simulink model "motor_kit_sim_20MHz"  (R2024a)
settings: Solver=VariableStepAuto  StartTime=0.0  StopTime=10*62.5E-6  RelTol=1e-3  EnableMultiTasking=on
PreLoadFcn:
  | setup_motor_kit_sim_20MHz;
InitFcn:
  | setup_motor_kit_sim_20MHz;
values from neighbouring files (symbols this model uses):
  DSPBASampleTime = 0.05e-6    (= 5e-08)    [setup_motor_kit_sim_20MHz.m]
  wordLength = 16    [setup_motor_kit_sim_20MHz.m]
undefined symbols (not defined in the file or in its folder): AdvDSPBChannelOutDisplay, dpoly, dspba_internal_get_channel_ports, evalAionMaskParam, latency, primtype, value, x
libraries: DSPBAPrim x317, DSPBAModelBus x25, DSPBABase x7, dspsrcs4 x3, simulink x3, DSPBAUtilities x1
(part 4 of 4)

== system motor_kit_sim_20MHz/MotorModel/MM_16fixed/MotorElectromagnetics_DSPBA_16fixed/Clarke_16fixed ==
  note: or:
      | (xb+xc) * (-0.5) + xa
  note: Transformation from 3-phase stator coil values to equivalent 2-phase values.
      | Scaling chosen so peak values remain the same.
      | Transformation equations:
      |
      | xAlpha = 2/3*(xa - 0.5*xb - 0.5*xc)
      | xBeta = 2/3*(sqrt(3)/2*xb - sqrt(3)/2*xc)
  xabc : Inport
  Add1 : DSPBAPrim/Add  primtype=add  nInputs=evalAionMaskParam(gcb,'value',1)  nOutputs=1  omode=Inherit via internal rule with word growth  otype=sfix(17)  scale=constScaleVoltage  rndmethod=Unbiased  factor=1  satmethod=Symmetric  shift_vec=[0 1 2 -1]  value=3  inPortNames=[' '; ' ';]  outPortNames=[' ']  dspbaimage=dspba_prim.svg  text=fprintf('+');  genFPC=off  floatRounding=correct  advOptions=[]  version=20240716
  Demux1 : Demux  Outputs=2
  Demux2 : Demux  Outputs=2
  Demux4 : Demux  Outputs=3
  Mux1 : Mux  Inputs=2
  Mux2 : Mux  Inputs=2
  Sub1 : DSPBAPrim/Sub  primtype=sub  nInputs=2  nOutputs=1  omode=Inherit via internal rule with word growth  otype=sfix(17)  scale=constScaleVoltage  rndmethod=Unbiased  factor=1  satmethod=Symmetric  shift_vec=[0 1 2 -1]  value=0  inPortNames=['+'; '-';]  outPortNames=[' ']  dspbaimage=dspba_prim.svg  text=fprintf('-');  floatRounding=correct  advOptions=[]  version=20240716
  Subsystem1 : Subsystem  mask{constVal=2/3}
      mask prompts: constVal "Gain"
      mask Display:
      | color('w');
      | set_param(gcb,'BackgroundColor','yellow');
      | fprintf('Gain\n%s', num2str(constVal));
      | port_label('input',1, 'a');
      | port_label('output',1,'b');
  Subsystem2 : Subsystem  mask{constVal=sqrt(3)/2}
      mask prompts: constVal "Gain"
      mask Display:
      | color('w');
      | set_param(gcb,'BackgroundColor','yellow');
      | fprintf('Gain\n%s', num2str(constVal));
      | port_label('input',1, 'a');
      | port_label('output',1,'b');
  Subsystem6 : Subsystem  mask{constVal=-1/2}
      mask prompts: constVal "Gain"
      mask Display:
      | color('w');
      | set_param(gcb,'BackgroundColor','yellow');
      | fprintf('Gain\n%s', num2str(constVal));
      | port_label('input',1, 'a');
      | port_label('output',1,'b');
  sfix16_En9_1 : DSPBAPrim/Convert  primtype=convert  nInputs=1  nOutputs=1  omode=Specify via dialog  otype=DataType  scale=constScaleVoltage  floatPrecision=float32_m23  rndmethod=Unbiased  factor=1  satmethod=Symmetric  shift_vec=[0 1 2 -1]  value=round([0:255]/17)  inPortNames=[' '; ' ';]  outPortNames=[' '; 'c']  dspbaimage=dspba_prim_wide.svg  text=fprintf('convert');  clipdetect=off  advOptions=[]  version=20240711
  sfix16_En9_2 : DSPBAPrim/Convert  primtype=convert  nInputs=1  nOutputs=1  omode=Specify via dialog  otype=DataType  scale=constScaleVoltage  floatPrecision=float32_m23  rndmethod=Unbiased  factor=1  satmethod=Symmetric  shift_vec=[0 1 2 -1]  value=round([0:255]/17)  inPortNames=[' '; ' ';]  outPortNames=[' '; 'c']  dspbaimage=dspba_prim_wide.svg  text=fprintf('convert');  clipdetect=off  advOptions=[]  version=20240711
  sfix16_En9_3 : DSPBAPrim/Convert  primtype=convert  nInputs=1  nOutputs=1  omode=Specify via dialog  otype=DataType  scale=constScaleVoltage  floatPrecision=float32_m23  rndmethod=Unbiased  factor=1  satmethod=Symmetric  shift_vec=[0 1 2 -1]  value=round([0:255]/17)  inPortNames=[' '; ' ';]  outPortNames=[' '; 'c']  dspbaimage=dspba_prim_wide.svg  text=fprintf('convert');  clipdetect=off  advOptions=[]  version=20240711
  xAlphaBeta : Outport
  wires:
  xabc/1 -> Demux4/1
  Demux4/2 -> Mux1/1  "xb"
  Demux4/3 -> Mux1/2  "xc"
  Mux1/1 -> Subsystem2/1(In1), Subsystem6/1(In1)
  Subsystem6/1(Out1) -> Demux1/1
  Demux4/1 -> Add1/1  "xa"
  Demux1/1 -> Add1/2  "-0.5*xb"
  Demux1/2 -> Add1/3  "-0.5*xc"
  Subsystem2/1(Out1) -> Demux2/1
  Demux2/1 -> Sub1/1  "(sqrt(3)/2)*xb"
  Demux2/2 -> Sub1/2  "(sqrt(3)/2)*xc"
  Mux2/1 -> Subsystem1/1(In1)
  Add1/1 -> sfix16_En9_2/1
  Sub1/1 -> sfix16_En9_1/1
  Subsystem1/1(Out1) -> sfix16_En9_3/1
  sfix16_En9_1/1 -> Mux2/2
  sfix16_En9_2/1 -> Mux2/1
  sfix16_En9_3/1 -> xAlphaBeta/1

== system motor_kit_sim_20MHz/MotorModel/MM_16fixed/MotorElectromagnetics_DSPBA_16fixed/ElectricalDynamicsDSPBA_16fixed ==
  vBemfAlpha_V : Inport
  vBemfBeta_V : Inport  Port=2
  vAlpha_V : Inport  Port=3
  vBeta_V : Inport  Port=4
  iAlpha_A_k_1 : Inport  Port=5
  iBeta_A_k_1 : Inport  Port=6
  SampleTime_s : Inport  Port=7
  Rphase_ohm : Inport  Port=8
  inv_Lphase_H : Inport  Port=9
  ElectricalDynamicsOnePhase_Alpha_DSPBA16fixed : Subsystem
  ElectricalDynamicsOnePhase_Beta_DSPBA16fixed : Subsystem
  SampleDelay : DSPBAPrim/SampleDelay  primtype=sampdelay  nInputs=1  nOutputs=1  omode=Inherit via internal rule  otype=sfix(16)  scale=2^-15  floatPrecision=float32_m23  rndmethod=Unbiased  factor=1  satmethod=Symmetric  shift_vec=[0 1 2 -1]  value=20  inPortNames=[' '; ' ';]  outPortNames=[' ']  dspbaimage=dspba_prim.svg  text=dpoly(1, eye(1,value+1), 'z')  flexible=off  slackgroup=0  augmented=0  version=20240711  advOptions=[]
  SampleDelay1 : DSPBAPrim/SampleDelay  primtype=sampdelay  nInputs=1  nOutputs=1  omode=Inherit via internal rule  otype=sfix(16)  scale=2^-15  floatPrecision=float32_m23  rndmethod=Unbiased  factor=1  satmethod=Symmetric  shift_vec=[0 1 2 -1]  value=20  inPortNames=[' '; ' ';]  outPortNames=[' ']  dspbaimage=dspba_prim.svg  text=dpoly(1, eye(1,value+1), 'z')  flexible=off  slackgroup=0  augmented=0  version=20240711  advOptions=[]
  Terminator : Terminator
  Terminator1 : Terminator
  diAlpha_dt_A_s : Outport
  diBeta_dt_A_s : Outport  Port=2
  iAlpha_A_k : Outport  Port=3
  iBeta_A_k : Outport  Port=4
  wires:
  vBeta_V/1 -> ElectricalDynamicsOnePhase_Beta_DSPBA16fixed/3(v_V)
  ElectricalDynamicsOnePhase_Beta_DSPBA16fixed/1(di_dt_A_s) -> diBeta_dt_A_s/1
  vBemfBeta_V/1 -> ElectricalDynamicsOnePhase_Beta_DSPBA16fixed/2(vBemf_V)
  SampleTime_s/1 -> ElectricalDynamicsOnePhase_Alpha_DSPBA16fixed/1(SampleTime_s), ElectricalDynamicsOnePhase_Beta_DSPBA16fixed/1(SampleTime_s)
  ElectricalDynamicsOnePhase_Alpha_DSPBA16fixed/2(i_A_k) -> SampleDelay/1, iAlpha_A_k/1
  ElectricalDynamicsOnePhase_Alpha_DSPBA16fixed/1(di_dt_A_s) -> diAlpha_dt_A_s/1
  Rphase_ohm/1 -> ElectricalDynamicsOnePhase_Beta_DSPBA16fixed/5(Rphase_ohm), ElectricalDynamicsOnePhase_Alpha_DSPBA16fixed/5(Rphase_ohm)
  inv_Lphase_H/1 -> ElectricalDynamicsOnePhase_Beta_DSPBA16fixed/6(inv_Lphase_H), ElectricalDynamicsOnePhase_Alpha_DSPBA16fixed/6(inv_Lphase_H)
  vAlpha_V/1 -> ElectricalDynamicsOnePhase_Alpha_DSPBA16fixed/3(v_V)
  vBemfAlpha_V/1 -> ElectricalDynamicsOnePhase_Alpha_DSPBA16fixed/2(vBemf_V)
  ElectricalDynamicsOnePhase_Beta_DSPBA16fixed/2(i_A_k) -> SampleDelay1/1, iBeta_A_k/1
  SampleDelay/1 -> ElectricalDynamicsOnePhase_Alpha_DSPBA16fixed/4(i_A_k_1)
  iAlpha_A_k_1/1 -> Terminator/1
  iBeta_A_k_1/1 -> Terminator1/1
  SampleDelay1/1 -> ElectricalDynamicsOnePhase_Beta_DSPBA16fixed/4(i_A_k_1)

== system motor_kit_sim_20MHz/MotorModel/MM_16fixed/MotorElectromagnetics_DSPBA_16fixed/Inv_Park_16fixed ==
  x_dq : Inport
  cos_phi_el : Inport  Port=2
  sin_phi_el : Inport  Port=3
  Add : DSPBAPrim/Add  primtype=add  nInputs=evalAionMaskParam(gcb,'value',1)  nOutputs=1  omode=Inherit via internal rule with word growth  otype=sfix(17)  scale=constScaleVoltage  rndmethod=Unbiased  factor=1  satmethod=Symmetric  shift_vec=[0 1 2 -1]  value=2  inPortNames=[' '; ' ';]  outPortNames=[' ']  dspbaimage=dspba_prim.svg  text=fprintf('+');  genFPC=off  floatRounding=correct  advOptions=[]  version=20240716
  Demux1 : Demux  Outputs=2
  Mult{1..4} (4 alike) : DSPBAPrim/Mult  primtype=mult  nInputs=2  nOutputs=1  omode=Inherit via internal rule  otype=DataType  scale=constScaleVoltage  floatPrecision=float32_m23  rndmethod=Unbiased  factor=1  satmethod=Symmetric  shift_vec=[0 1 2 -1]  value=0  inPortNames=[' '; ' ';]  outPortNames=[' ']  dspbaimage=dspba_prim.svg  text=fprintf('X');  floatRounding=correct  advOptions=[]  version=20240711
  Mux2 : Mux  Inputs=2
  Sub1 : DSPBAPrim/Sub  primtype=sub  nInputs=2  nOutputs=1  omode=Inherit via internal rule with word growth  otype=sfix(17)  scale=constScaleVoltage  rndmethod=Unbiased  factor=1  satmethod=Symmetric  shift_vec=[0 1 2 -1]  value=0  inPortNames=['+'; '-';]  outPortNames=[' ']  dspbaimage=dspba_prim.svg  text=fprintf('-');  floatRounding=correct  advOptions=[]  version=20240716
  sfix16_{0..5} (6 alike) : DSPBAPrim/Convert  primtype=convert  nInputs=1  nOutputs=1  omode=Specify via dialog  otype=DataType  scale=constScaleVoltage  floatPrecision=float32_m23  rndmethod=Unbiased  factor=1  satmethod=Symmetric  shift_vec=[0 1 2 -1]  value=round([0:255]/17)  inPortNames=[' '; ' ';]  outPortNames=[' '; 'c']  dspbaimage=dspba_prim_wide.svg  text=fprintf('convert');  clipdetect=off  advOptions=[]  version=20240711
  x_AlphaBeta : Outport
  wires:
  sin_phi_el/1 -> Mult2/2, Mult3/2
  Mult4/1 -> sfix16_3/1
  Mult3/1 -> sfix16_2/1
  Mult2/1 -> sfix16_1/1
  Mult1/1 -> sfix16_0/1
  Add/1 -> sfix16_5/1
  Sub1/1 -> sfix16_4/1
  Demux1/2 -> Mult2/1, Mult4/1
  Demux1/1 -> Mult1/1, Mult3/1
  x_dq/1 -> Demux1/1
  cos_phi_el/1 -> Mult1/2, Mult4/2
  Mux2/1 -> x_AlphaBeta/1
  sfix16_0/1 -> Sub1/1
  sfix16_1/1 -> Sub1/2
  sfix16_2/1 -> Add/1
  sfix16_3/1 -> Add/2
  sfix16_4/1 -> Mux2/1
  sfix16_5/1 -> Mux2/2

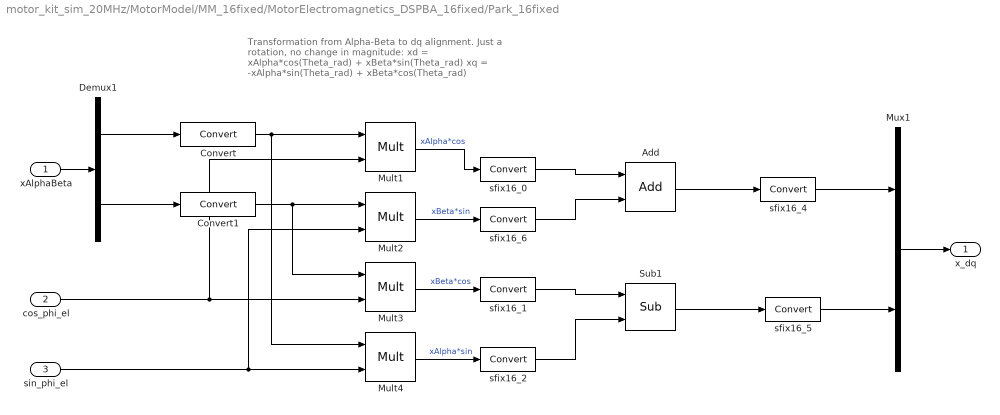
== system motor_kit_sim_20MHz/MotorModel/MM_16fixed/MotorElectromagnetics_DSPBA_16fixed/Park_16fixed ==
  note: Transformation from Alpha-Beta to dq alignment.
      | Just a rotation, no change in magnitude:
      |
      | xd = xAlpha*cos(Theta_rad) + xBeta*sin(Theta_rad)
      | xq = -xAlpha*sin(Theta_rad) + xBeta*cos(Theta_rad)
  xAlphaBeta : Inport
  cos_phi_el : Inport  Port=2
  sin_phi_el : Inport  Port=3
  Add : DSPBAPrim/Add  primtype=add  nInputs=evalAionMaskParam(gcb,'value',1)  nOutputs=1  omode=Inherit via internal rule with word growth  otype=sfix(17)  scale=constScaleCurrent  rndmethod=Unbiased  factor=1  satmethod=Symmetric  shift_vec=[0 1 2 -1]  value=2  inPortNames=[' '; ' ';]  outPortNames=[' ']  dspbaimage=dspba_prim.svg  text=fprintf('+');  genFPC=off  floatRounding=correct  advOptions=[]  version=20240716
  Convert : DSPBAPrim/Convert  primtype=convert  nInputs=1  nOutputs=1  omode=Specify via dialog  otype=sfix(27)  scale=2^-19  floatPrecision=float32_m23  rndmethod=Biased  factor=1  satmethod=None  shift_vec=[0 1 2 -1]  value=round([0:255]/17)  inPortNames=[' '; ' ';]  outPortNames=[' '; 'c']  dspbaimage=dspba_prim_wide.svg  text=fprintf('convert');  clipdetect=off  advOptions=[]  version=20240711
  Convert1 : DSPBAPrim/Convert  primtype=convert  nInputs=1  nOutputs=1  omode=Specify via dialog  otype=sfix(27)  scale=2^-19  floatPrecision=float32_m23  rndmethod=Biased  factor=1  satmethod=None  shift_vec=[0 1 2 -1]  value=round([0:255]/17)  inPortNames=[' '; ' ';]  outPortNames=[' '; 'c']  dspbaimage=dspba_prim_wide.svg  text=fprintf('convert');  clipdetect=off  advOptions=[]  version=20240711
  Demux1 : Demux  Outputs=2
  Mult{1..4} (4 alike) : DSPBAPrim/Mult  primtype=mult  nInputs=2  nOutputs=1  omode=Inherit via internal rule  otype=DataType  scale=constScaleCurrent  floatPrecision=float32_m23  rndmethod=Unbiased  factor=1  satmethod=Symmetric  shift_vec=[0 1 2 -1]  value=0  inPortNames=[' '; ' ';]  outPortNames=[' ']  dspbaimage=dspba_prim.svg  text=fprintf('X');  floatRounding=correct  advOptions=[]  version=20240711
  Mux1 : Mux  Inputs=2
  Sub1 : DSPBAPrim/Sub  primtype=sub  nInputs=2  nOutputs=1  omode=Inherit via internal rule with word growth  otype=sfix(17)  scale=constScaleCurrent  rndmethod=Unbiased  factor=1  satmethod=Symmetric  shift_vec=[0 1 2 -1]  value=0  inPortNames=['+'; '-';]  outPortNames=[' ']  dspbaimage=dspba_prim.svg  text=fprintf('-');  floatRounding=correct  advOptions=[]  version=20240716
  sfix16_{0..2,6} (4 alike) : DSPBAPrim/Convert  primtype=convert  nInputs=1  nOutputs=1  omode=Specify via dialog  otype=sfix(43)  scale=2^-33  floatPrecision=float32_m23  rndmethod=Unbiased  factor=1  satmethod=Symmetric  shift_vec=[0 1 2 -1]  value=round([0:255]/17)  inPortNames=[' '; ' ';]  outPortNames=[' '; 'c']  dspbaimage=dspba_prim_wide.svg  text=fprintf('convert');  clipdetect=off  advOptions=[]  version=20240711
  sfix16_4 : DSPBAPrim/Convert  primtype=convert  nInputs=1  nOutputs=1  omode=Specify via dialog  otype=DataType_dq  scale=constScale_dq  floatPrecision=float32_m23  rndmethod=Unbiased  factor=1  satmethod=Symmetric  shift_vec=[0 1 2 -1]  value=round([0:255]/17)  inPortNames=[' '; ' ';]  outPortNames=[' '; 'c']  dspbaimage=dspba_prim_wide.svg  text=fprintf('convert');  clipdetect=off  advOptions=[]  version=20240711
  sfix16_5 : DSPBAPrim/Convert  primtype=convert  nInputs=1  nOutputs=1  omode=Specify via dialog  otype=DataType_dq  scale=constScale_dq  floatPrecision=float32_m23  rndmethod=Unbiased  factor=1  satmethod=Symmetric  shift_vec=[0 1 2 -1]  value=round([0:255]/17)  inPortNames=[' '; ' ';]  outPortNames=[' '; 'c']  dspbaimage=dspba_prim_wide.svg  text=fprintf('convert');  clipdetect=off  advOptions=[]  version=20240711
  x_dq : Outport
  wires:
  cos_phi_el/1 -> Mult3/2, Mult1/2
  sin_phi_el/1 -> Mult4/2, Mult2/2
  Mux1/1 -> x_dq/1
  Mult1/1 -> sfix16_0/1  "xAlpha*cos"
  Mult2/1 -> sfix16_6/1  "xBeta*sin"
  Mult4/1 -> sfix16_2/1  "xAlpha*sin"
  Mult3/1 -> sfix16_1/1  "xBeta*cos"
  xAlphaBeta/1 -> Demux1/1
  sfix16_0/1 -> Add/1
  sfix16_6/1 -> Add/2
  sfix16_1/1 -> Sub1/1
  sfix16_2/1 -> Sub1/2
  Sub1/1 -> sfix16_5/1
  Add/1 -> sfix16_4/1
  sfix16_4/1 -> Mux1/1
  sfix16_5/1 -> Mux1/2
  Demux1/1 -> Convert/1
  Convert/1 -> Mult4/1, Mult1/1
  Demux1/2 -> Convert1/1
  Convert1/1 -> Mult3/1, Mult2/1

== system motor_kit_sim_20MHz/MotorModel/MM_16fixed/MotorElectromagnetics_DSPBA_16fixed/Park_16fixed1 ==
  note: Transformation from Alpha-Beta to dq alignment.
      | Just a rotation, no change in magnitude:
      |
      | xd = xAlpha*cos(Theta_rad) + xBeta*sin(Theta_rad)
      | xq = -xAlpha*sin(Theta_rad) + xBeta*cos(Theta_rad)
  xAlphaBeta : Inport
  cos_phi_el : Inport  Port=2
  sin_phi_el : Inport  Port=3
  Add : DSPBAPrim/Add  primtype=add  nInputs=evalAionMaskParam(gcb,'value',1)  nOutputs=1  omode=Inherit via internal rule with word growth  otype=sfix(17)  scale=constScaleCurrentDerivative  rndmethod=Unbiased  factor=1  satmethod=Symmetric  shift_vec=[0 1 2 -1]  value=2  inPortNames=[' '; ' ';]  outPortNames=[' ']  dspbaimage=dspba_prim.svg  text=fprintf('+');  genFPC=off  floatRounding=correct  advOptions=[]  version=20240716
  Demux1 : Demux  Outputs=2
  Mult{1..4} (4 alike) : DSPBAPrim/Mult  primtype=mult  nInputs=2  nOutputs=1  omode=Inherit via internal rule  otype=DataType  scale=constScaleCurrentDerivative  floatPrecision=float32_m23  rndmethod=Unbiased  factor=1  satmethod=Symmetric  shift_vec=[0 1 2 -1]  value=0  inPortNames=[' '; ' ';]  outPortNames=[' ']  dspbaimage=dspba_prim.svg  text=fprintf('X');  floatRounding=correct  advOptions=[]  version=20240711
  Mux1 : Mux  Inputs=2
  Sub1 : DSPBAPrim/Sub  primtype=sub  nInputs=2  nOutputs=1  omode=Inherit via internal rule with word growth  otype=sfix(17)  scale=constScaleCurrentDerivative  rndmethod=Unbiased  factor=1  satmethod=Symmetric  shift_vec=[0 1 2 -1]  value=0  inPortNames=['+'; '-';]  outPortNames=[' ']  dspbaimage=dspba_prim.svg  text=fprintf('-');  floatRounding=correct  advOptions=[]  version=20240716
  sfix16_En{1..4} (4 alike) : DSPBAPrim/Convert  primtype=convert  nInputs=1  nOutputs=1  omode=Specify via dialog  otype=sfix(32)  scale=2^-15  floatPrecision=float32_m23  rndmethod=Unbiased  factor=1  satmethod=Symmetric  shift_vec=[0 1 2 -1]  value=round([0:255]/17)  inPortNames=[' '; ' ';]  outPortNames=[' '; 'c']  dspbaimage=dspba_prim_wide.svg  text=fprintf('convert');  clipdetect=off  advOptions=[]  version=20240711
  x_dq : Outport
  wires:
  cos_phi_el/1 -> Mult3/2, Mult1/2
  Demux1/2 -> Mult3/1, Mult2/1
  sin_phi_el/1 -> Mult4/2, Mult2/2
  Mux1/1 -> x_dq/1
  Mult1/1 -> sfix16_En3/1
  Mult2/1 -> sfix16_En1/1
  Demux1/1 -> Mult4/1, Mult1/1
  Mult4/1 -> sfix16_En4/1
  Mult3/1 -> sfix16_En2/1
  xAlphaBeta/1 -> Demux1/1
  Add/1 -> Mux1/1
  Sub1/1 -> Mux1/2
  sfix16_En3/1 -> Add/1
  sfix16_En1/1 -> Add/2
  sfix16_En2/1 -> Sub1/1
  sfix16_En4/1 -> Sub1/2

== system motor_kit_sim_20MHz/MotorModel/MM_16fixed/MotorElectromagnetics_DSPBA_16fixed/Park_16fixed2 ==
  note: Transformation from Alpha-Beta to dq alignment.
      | Just a rotation, no change in magnitude:
      |
      | xd = xAlpha*cos(Theta_rad) + xBeta*sin(Theta_rad)
      | xq = -xAlpha*sin(Theta_rad) + xBeta*cos(Theta_rad)
  xAlphaBeta : Inport
  cos_phi_el : Inport  Port=2
  sin_phi_el : Inport  Port=3
  Add : DSPBAPrim/Add  primtype=add  nInputs=evalAionMaskParam(gcb,'value',1)  nOutputs=1  omode=Inherit via internal rule with word growth  otype=sfix(17)  scale=constScaleVoltage  rndmethod=Unbiased  factor=1  satmethod=Symmetric  shift_vec=[0 1 2 -1]  value=2  inPortNames=[' '; ' ';]  outPortNames=[' ']  dspbaimage=dspba_prim.svg  text=fprintf('+');  genFPC=off  floatRounding=correct  advOptions=[]  version=20240716
  Demux1 : Demux  Outputs=2
  Mult{1..4} (4 alike) : DSPBAPrim/Mult  primtype=mult  nInputs=2  nOutputs=1  omode=Inherit via internal rule  otype=DataType  scale=constScaleVoltage  floatPrecision=float32_m23  rndmethod=Unbiased  factor=1  satmethod=Symmetric  shift_vec=[0 1 2 -1]  value=0  inPortNames=[' '; ' ';]  outPortNames=[' ']  dspbaimage=dspba_prim.svg  text=fprintf('X');  floatRounding=correct  advOptions=[]  version=20240711
  Mux1 : Mux  Inputs=2
  Sub1 : DSPBAPrim/Sub  primtype=sub  nInputs=2  nOutputs=1  omode=Inherit via internal rule with word growth  otype=sfix(17)  scale=constScaleVoltage  rndmethod=Unbiased  factor=1  satmethod=Symmetric  shift_vec=[0 1 2 -1]  value=0  inPortNames=['+'; '-';]  outPortNames=[' ']  dspbaimage=dspba_prim.svg  text=fprintf('-');  floatRounding=correct  advOptions=[]  version=20240716
  sfix16_{0..5} (6 alike) : DSPBAPrim/Convert  primtype=convert  nInputs=1  nOutputs=1  omode=Specify via dialog  otype=DataType  scale=constScaleVoltage  floatPrecision=float32_m23  rndmethod=Unbiased  factor=1  satmethod=Symmetric  shift_vec=[0 1 2 -1]  value=round([0:255]/17)  inPortNames=[' '; ' ';]  outPortNames=[' '; 'c']  dspbaimage=dspba_prim_wide.svg  text=fprintf('convert');  clipdetect=off  advOptions=[]  version=20240711
  x_dq : Outport
  wires:
  xAlphaBeta/1 -> Demux1/1
  Mult3/1 -> sfix16_2/1
  Mult4/1 -> sfix16_3/1
  Demux1/1 -> Mult1/1, Mult4/1
  Mult2/1 -> sfix16_1/1
  Mult1/1 -> sfix16_0/1
  Add/1 -> sfix16_4/1
  Sub1/1 -> sfix16_5/1
  Mux1/1 -> x_dq/1
  sin_phi_el/1 -> Mult4/2, Mult2/2
  Demux1/2 -> Mult2/1, Mult3/1
  cos_phi_el/1 -> Mult3/2, Mult1/2
  sfix16_0/1 -> Add/1
  sfix16_1/1 -> Add/2
  sfix16_2/1 -> Sub1/1
  sfix16_3/1 -> Sub1/2
  sfix16_4/1 -> Mux1/1
  sfix16_5/1 -> Mux1/2

== system motor_kit_sim_20MHz/MotorModel/MM_16fixed/MotorElectromagnetics_DSPBA_16fixed/inv_Clarke_16fixed ==
  note: Transformation from equivalent Alpha-Beta 2-phase stator-based values to original 3-phase stator coil values.
      | Scaling chosen so peak values remain the same.
      | Transformation equations:
      |
      | xa = xAlpha
      | xb = -0.5*xAlpha + 0.5*sqrt(3)*xBeta
      | xc = -0.5*xAlpha - 0.5*sqrt(3)*xBeta
  xAlphaBeta : Inport
  Add : DSPBAPrim/Add  primtype=add  nInputs=evalAionMaskParam(gcb,'value',1)  nOutputs=1  omode=Inherit via internal rule with word growth  otype=sfix(17)  scale=constScaleCurrent  rndmethod=Unbiased  factor=1  satmethod=Symmetric  shift_vec=[0 1 2 -1]  value=2  inPortNames=[' '; ' ';]  outPortNames=[' ']  dspbaimage=dspba_prim.svg  text=fprintf('+');  genFPC=off  floatRounding=correct  advOptions=[]  version=20240716
  Demux1 : Demux  Outputs=2
  Mux1 : Mux  Inputs=3
  Sub3 : DSPBAPrim/Sub  primtype=sub  nInputs=2  nOutputs=1  omode=Inherit via internal rule with word growth  otype=sfix(17)  scale=constScaleCurrent  rndmethod=Unbiased  factor=1  satmethod=Symmetric  shift_vec=[0 1 2 -1]  value=0  inPortNames=['+'; '-';]  outPortNames=[' ']  dspbaimage=dspba_prim.svg  text=fprintf('-');  floatRounding=correct  advOptions=[]  version=20240716
  Subsystem1 : Subsystem  mask{constVal=-1/2}
      mask prompts: constVal "Gain"
      mask Display:
      | color('w');
      | set_param(gcb,'BackgroundColor','yellow');
      | fprintf('Gain\n%s', num2str(constVal));
      | port_label('input',1, 'a');
      | port_label('output',1,'b');
  Subsystem4 : Subsystem  mask{constVal=sqrt(3)}
      mask prompts: constVal "Gain"
      mask Display:
      | color('w');
      | set_param(gcb,'BackgroundColor','yellow');
      | fprintf('sqrt(3)\n', num2str(constVal));
      | port_label('input', 1, 'a');
      | port_label('output', 1, 'b');
  Subsystem5 : Subsystem  mask{constVal=1/2}
      mask prompts: constVal "Gain"
      mask Display:
      | color('w');
      | set_param(gcb,'BackgroundColor','yellow');
      | fprintf('Gain\n%s', num2str(constVal));
      | port_label('input',1, 'a');
      | port_label('output',1,'b');
  sfix16_1 : DSPBAPrim/Convert  primtype=convert  nInputs=1  nOutputs=1  omode=Specify via dialog  otype=DataType  scale=constScaleCurrent  floatPrecision=float32_m23  rndmethod=Unbiased  factor=1  satmethod=Symmetric  shift_vec=[0 1 2 -1]  value=round([0:255]/17)  inPortNames=[' '; ' ';]  outPortNames=[' '; 'c']  dspbaimage=dspba_prim_wide.svg  text=fprintf('convert');  clipdetect=off  advOptions=[]  version=20240711
  sfix16_2 : DSPBAPrim/Convert  primtype=convert  nInputs=1  nOutputs=1  omode=Specify via dialog  otype=DataType  scale=constScaleCurrent  floatPrecision=float32_m23  rndmethod=Unbiased  factor=1  satmethod=Symmetric  shift_vec=[0 1 2 -1]  value=round([0:255]/17)  inPortNames=[' '; ' ';]  outPortNames=[' '; 'c']  dspbaimage=dspba_prim_wide.svg  text=fprintf('convert');  clipdetect=off  advOptions=[]  version=20240711
  sfix16_4 : DSPBAPrim/Convert  primtype=convert  nInputs=1  nOutputs=1  omode=Specify via dialog  otype=DataType  scale=constScaleCurrent  floatPrecision=float32_m23  rndmethod=Unbiased  factor=1  satmethod=Symmetric  shift_vec=[0 1 2 -1]  value=round([0:255]/17)  inPortNames=[' '; ' ';]  outPortNames=[' '; 'c']  dspbaimage=dspba_prim_wide.svg  text=fprintf('convert');  clipdetect=off  advOptions=[]  version=20240711
  xabc : Outport
  wires:
  Subsystem5/1(Out1) -> Subsystem4/1(In1)
  Demux1/2 -> Subsystem5/1(In1)
  Demux1/1 -> sfix16_2/1, Subsystem1/1(In1)  "xa"
  Add/1 -> sfix16_1/1  "xb"
  Mux1/1 -> xabc/1
  Subsystem4/1(Out1) -> Sub3/2, Add/1
  Subsystem1/1(Out1) -> Sub3/1, Add/2
  xAlphaBeta/1 -> Demux1/1
  Sub3/1 -> sfix16_4/1  "xc"
  sfix16_1/1 -> Mux1/2
  sfix16_4/1 -> Mux1/3
  sfix16_2/1 -> Mux1/1

== system motor_kit_sim_20MHz/MotorModel/MM_16fixed/MotorElectromagnetics_DSPBA_16fixed/sine_cosine_16fixed ==
  note: 2 sine blocks are used to calculate sine and cosine.
      | This allows the ALU folder to reduce resource usage.
  pole pairs : Inport
  theta mechanical one turn : Inport  Port=2
  Const : DSPBAPrim/Const  primtype=const  nInputs=0  nOutputs=1  omode=Specify via dialog  otype=ufix(2)  scale=2^-0  floatPrecision=float26_m17  rndmethod=Unbiased  factor=1  satmethod=Symmetric  shift_vec=[0 1 2 -1]  value=2  inPortNames=['+'; '+';]  outPortNames=[' ']  dspbaimage=dspba_prim.svg  text=fprintf('%s', num2str(value));  warnSaturation=on  version=20240711  SampleTime=inf
  Const1 : DSPBAPrim/Const  primtype=const  nInputs=0  nOutputs=1  omode=Specify via dialog  otype=ufix(16)  scale=2^-14  floatPrecision=float26_m17  rndmethod=Unbiased  factor=1  satmethod=Symmetric  shift_vec=[0 1 2 -1]  value=1/2  inPortNames=['+'; '+';]  outPortNames=[' ']  dspbaimage=dspba_prim.svg  text=fprintf('%s', num2str(value));  warnSaturation=on  version=20240711  SampleTime=inf
  Convert : DSPBAPrim/Convert  primtype=convert  nInputs=1  nOutputs=1  omode=Specify via dialog  otype=ufix(18)  scale=2^-18  floatPrecision=float32_m23  rndmethod=Biased  factor=1  satmethod=None  shift_vec=[0 1 2 -1]  value=round([0:255]/17)  inPortNames=[' '; ' ';]  outPortNames=[' '; 'c']  dspbaimage=dspba_prim_wide.svg  text=fprintf('convert');  clipdetect=off  advOptions=[]  version=20240711
  Mult1 : DSPBAPrim/Mult  primtype=mult  nInputs=2  nOutputs=1  omode=Inherit via internal rule  otype=DataType  scale=2^-14  floatPrecision=float32_m23  rndmethod=Unbiased  factor=1  satmethod=Symmetric  shift_vec=[0 1 2 -1]  value=0  inPortNames=[' '; ' ';]  outPortNames=[' ']  dspbaimage=dspba_prim.svg  text=fprintf('X');  floatRounding=correct  advOptions=[]  version=20240711
  Mult2 : DSPBAPrim/Mult  primtype=mult  nInputs=2  nOutputs=1  omode=Inherit via internal rule  otype=ufix(16)  scale=2^-14  floatPrecision=float32_m23  rndmethod=Unbiased  factor=1  satmethod=Symmetric  shift_vec=[0 1 2 -1]  value=0  inPortNames=[' '; ' ';]  outPortNames=[' ']  dspbaimage=dspba_prim.svg  text=fprintf('X');  floatRounding=correct  advOptions=[]  version=20240711
  Sub : DSPBAPrim/Sub  primtype=sub  nInputs=2  nOutputs=1  omode=Inherit via internal rule with word growth  otype=ufix(17)  scale=2^-14  rndmethod=Unbiased  factor=1  satmethod=Symmetric  shift_vec=[0 1 2 -1]  value=0  inPortNames=['+'; '-';]  outPortNames=[' ']  dspbaimage=dspba_prim.svg  text=fprintf('-');  floatRounding=correct  advOptions=[]  version=20240716
  Trig1 : DSPBAPrim/Trig  primtype=trigfunc  nInputs=1  nOutputs=1  omode=Inherit via internal rule  otype=sfix(16)  scale=2^-15  rndmethod=Unbiased  factor=1  satmethod=Symmetric  shift_vec=[0 1 2 -1]  value=round([0:255]/17)  inPortNames=[' '; ' ';]  outPortNames=[' ']  dspbaimage=dspba_prim_float.svg  text=fprintf('sin(a)');  functionExpr=sin(pi*x)  advOptions=[]  version=20240715
  Trig2 : DSPBAPrim/Trig  primtype=trigfunc  nInputs=1  nOutputs=1  omode=Inherit via internal rule  otype=sfix(16)  scale=2^-15  rndmethod=Unbiased  factor=1  satmethod=Symmetric  shift_vec=[0 1 2 -1]  value=round([0:255]/17)  inPortNames=[' '; ' ';]  outPortNames=[' ']  dspbaimage=dspba_prim_float.svg  text=fprintf('sin(a)');  functionExpr=sin(pi*x)  advOptions=[]  version=20240715
  modulus : Subsystem
  sfix16_En13_0 : DSPBAPrim/Convert  primtype=convert  nInputs=1  nOutputs=1  omode=Specify via dialog  otype=DataTypeU  scale=constScaleSinCos  floatPrecision=float32_m23  rndmethod=Unbiased  factor=1  satmethod=None  shift_vec=[0 1 2 -1]  value=round([0:255]/17)  inPortNames=[' '; ' ';]  outPortNames=[' '; 'c']  dspbaimage=dspba_prim_wide.svg  text=fprintf('convert');  clipdetect=off  advOptions=[]  version=20240711
  sfix16_En13_2 : DSPBAPrim/Convert  primtype=convert  nInputs=1  nOutputs=1  omode=Specify via dialog  otype=DataTypeU  scale=constScaleSinCos  floatPrecision=float32_m23  rndmethod=Unbiased  factor=1  satmethod=None  shift_vec=[0 1 2 -1]  value=round([0:255]/17)  inPortNames=[' '; ' ';]  outPortNames=[' '; 'c']  dspbaimage=dspba_prim_wide.svg  text=fprintf('convert');  clipdetect=off  advOptions=[]  version=20240711
  sfix16_En14 : DSPBAPrim/Convert  primtype=convert  nInputs=1  nOutputs=1  omode=Specify via dialog  otype=DataType  scale=constScaleTrig  floatPrecision=float32_m23  rndmethod=Unbiased  factor=1  satmethod=Symmetric  shift_vec=[0 1 2 -1]  value=round([0:255]/17)  inPortNames=[' '; ' ';]  outPortNames=[' '; 'c']  dspbaimage=dspba_prim_wide.svg  text=fprintf('convert');  clipdetect=off  advOptions=[]  version=20240711
  sine : Outport
  cosine : Outport  Port=2
  wires:
  modulus/1(Out1) -> Mult2/1
  Mult1/1 -> sfix16_En14/1
  Const/1 -> Mult2/2
  theta mechanical one turn/1 -> Convert/1
  Const1/1 -> Sub/1
  pole pairs/1 -> Mult1/1
  Trig1/1 -> sine/1
  Mult2/1 -> sfix16_En13_0/1
  sfix16_En14/1 -> modulus/1(In1)
  sfix16_En13_0/1 -> Trig1/1, Sub/2
  Sub/1 -> sfix16_En13_2/1
  Trig2/1 -> cosine/1
  sfix16_En13_2/1 -> Trig2/1
  Convert/1 -> Mult1/2

== system motor_kit_sim_20MHz/MotorModel/MM_16fixed/MotorInertia_DSPBA_16fixed/Subsystem3 ==
  In1 : Inport
  Const : DSPBAPrim/Const  primtype=const  nInputs=0  nOutputs=1  omode=Specify via dialog  otype=ufix(16)  scale=2^-18  floatPrecision=float32_m23  rndmethod=Unbiased  factor=1  satmethod=Symmetric  shift_vec=[0 1 2 -1]  value=constVal  inPortNames=['+'; '+';]  outPortNames=[' ']  dspbaimage=dspba_prim.svg  text=fprintf('%s', num2str(value));  warnSaturation=on  version=20240711  SampleTime=inf
  Mult : DSPBAPrim/Mult  primtype=mult  nInputs=2  nOutputs=1  omode=Inherit via internal rule  otype=sfix(32)  scale=2^-28  floatPrecision=float32_m23  rndmethod=Unbiased  factor=1  satmethod=Symmetric  shift_vec=[0 1 2 -1]  value=0  inPortNames=[' '; ' ';]  outPortNames=[' ']  dspbaimage=dspba_prim.svg  text=fprintf('X');  floatRounding=correct  advOptions=[]  version=20240711
  Out1 : Outport
  wires:
  Mult/1 -> Out1/1
  In1/1 -> Mult/1
  Const/1 -> Mult/2

== system motor_kit_sim_20MHz/MotorModel/MM_16fixed/MotorElectromagnetics_DSPBA_16fixed/Clarke_16fixed/Subsystem1 ==
  In1 : Inport
  Const3 : DSPBAPrim/Const  primtype=const  nInputs=0  nOutputs=1  omode=Specify via dialog  otype=DataType  scale=2^-15  floatPrecision=float32_m23  rndmethod=Unbiased  factor=1  satmethod=Symmetric  shift_vec=[0 1 2 -1]  value=constVal  inPortNames=['+'; '+';]  outPortNames=[' ']  dspbaimage=dspba_prim.svg  text=fprintf('%s', num2str(value));  warnSaturation=on  version=20240711  SampleTime=inf
  Mult1 : DSPBAPrim/Mult  primtype=mult  nInputs=2  nOutputs=1  omode=Inherit via internal rule  otype=DataType  scale=constScaleVoltage  floatPrecision=float32_m23  rndmethod=Unbiased  factor=1  satmethod=Symmetric  shift_vec=[0 1 2 -1]  value=0  inPortNames=[' '; ' ';]  outPortNames=[' ']  dspbaimage=dspba_prim.svg  text=fprintf('X');  floatRounding=correct  advOptions=[]  version=20240711
  Out1 : Outport
  wires:
  In1/1 -> Mult1/1
  Mult1/1 -> Out1/1
  Const3/1 -> Mult1/2

== system motor_kit_sim_20MHz/MotorModel/MM_16fixed/MotorElectromagnetics_DSPBA_16fixed/Clarke_16fixed/Subsystem2 ==
  In1 : Inport
  Const3 : DSPBAPrim/Const  primtype=const  nInputs=0  nOutputs=1  omode=Specify via dialog  otype=DataType  scale=2^-15  floatPrecision=float32_m23  rndmethod=Unbiased  factor=1  satmethod=Symmetric  shift_vec=[0 1 2 -1]  value=constVal  inPortNames=['+'; '+';]  outPortNames=[' ']  dspbaimage=dspba_prim.svg  text=fprintf('%s', num2str(value));  warnSaturation=on  version=20240711  SampleTime=inf
  Mult1 : DSPBAPrim/Mult  primtype=mult  nInputs=2  nOutputs=1  omode=Inherit via internal rule  otype=DataType  scale=constScaleVoltage  floatPrecision=float32_m23  rndmethod=Unbiased  factor=1  satmethod=Symmetric  shift_vec=[0 1 2 -1]  value=0  inPortNames=[' '; ' ';]  outPortNames=[' ']  dspbaimage=dspba_prim.svg  text=fprintf('X');  floatRounding=correct  advOptions=[]  version=20240711
  Out1 : Outport
  wires:
  In1/1 -> Mult1/1
  Mult1/1 -> Out1/1
  Const3/1 -> Mult1/2

== system motor_kit_sim_20MHz/MotorModel/MM_16fixed/MotorElectromagnetics_DSPBA_16fixed/Clarke_16fixed/Subsystem6 ==
  In1 : Inport
  Const3 : DSPBAPrim/Const  primtype=const  nInputs=0  nOutputs=1  omode=Specify via dialog  otype=DataType  scale=2^-15  floatPrecision=float32_m23  rndmethod=Unbiased  factor=1  satmethod=Symmetric  shift_vec=[0 1 2 -1]  value=constVal  inPortNames=['+'; '+';]  outPortNames=[' ']  dspbaimage=dspba_prim.svg  text=fprintf('%s', num2str(value));  warnSaturation=on  version=20240711  SampleTime=inf
  Mult1 : DSPBAPrim/Mult  primtype=mult  nInputs=2  nOutputs=1  omode=Inherit via internal rule  otype=DataType  scale=constScaleVoltage  floatPrecision=float32_m23  rndmethod=Unbiased  factor=1  satmethod=Symmetric  shift_vec=[0 1 2 -1]  value=0  inPortNames=[' '; ' ';]  outPortNames=[' ']  dspbaimage=dspba_prim.svg  text=fprintf('X');  floatRounding=correct  advOptions=[]  version=20240711
  Out1 : Outport
  wires:
  Const3/1 -> Mult1/2
  Mult1/1 -> Out1/1
  In1/1 -> Mult1/1

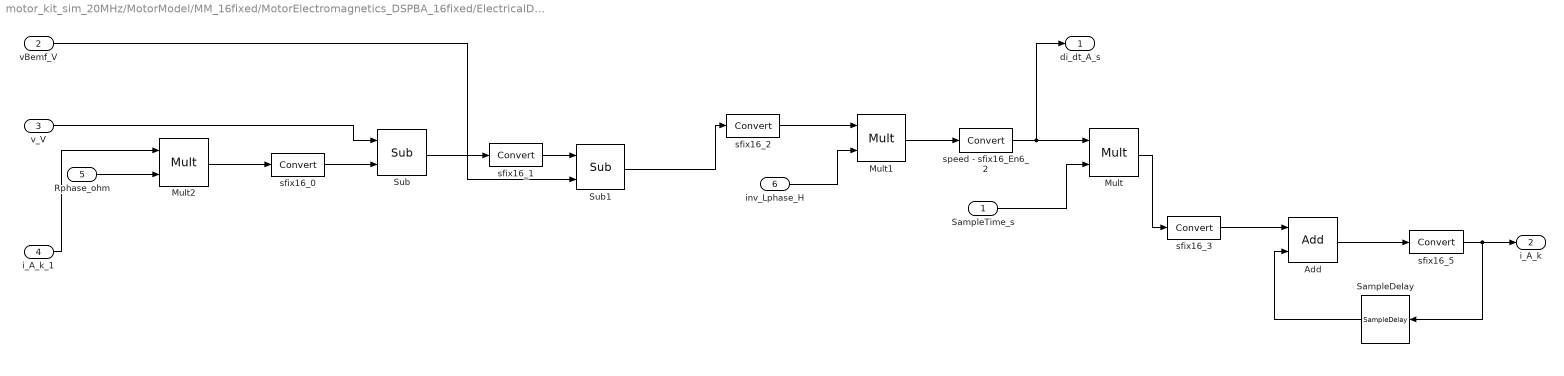
== system motor_kit_sim_20MHz/MotorModel/MM_16fixed/MotorElectromagnetics_DSPBA_16fixed/ElectricalDynamicsDSPBA_16fixed/ElectricalDynamicsOnePhase_Alpha_DSPBA16fixed ==
  SampleTime_s : Inport
  vBemf_V : Inport  Port=2
  v_V : Inport  Port=3
  i_A_k_1 : Inport  Port=4
  Rphase_ohm : Inport  Port=5
  inv_Lphase_H : Inport  Port=6
  Add : DSPBAPrim/Add  primtype=add  nInputs=evalAionMaskParam(gcb,'value',1)  nOutputs=1  omode=Inherit via internal rule with word growth  otype=sfix(17)  scale=constScaleCurrent  rndmethod=Unbiased  factor=1  satmethod=Symmetric  shift_vec=[0 1 2 -1]  value=2  inPortNames=[' '; ' ';]  outPortNames=[' ']  dspbaimage=dspba_prim.svg  text=fprintf('+');  genFPC=off  floatRounding=correct  advOptions=[]  version=20240716
  Mult : DSPBAPrim/Mult  primtype=mult  nInputs=2  nOutputs=1  omode=Inherit via internal rule  otype=sfix(32)  scale=2^-18  floatPrecision=float32_m23  rndmethod=Unbiased  factor=1  satmethod=Symmetric  shift_vec=[0 1 2 -1]  value=0  inPortNames=[' '; ' ';]  outPortNames=[' ']  dspbaimage=dspba_prim.svg  text=fprintf('X');  floatRounding=correct  advOptions=[]  version=20240711
  Mult1 : DSPBAPrim/Mult  primtype=mult  nInputs=2  nOutputs=1  omode=Inherit via internal rule  otype=DataType  scale=constScaleCurrentDerivative  floatPrecision=float32_m23  rndmethod=Unbiased  factor=1  satmethod=Symmetric  shift_vec=[0 1 2 -1]  value=0  inPortNames=[' '; ' ';]  outPortNames=[' ']  dspbaimage=dspba_prim.svg  text=fprintf('X');  floatRounding=correct  advOptions=[]  version=20240711
  Mult2 : DSPBAPrim/Mult  primtype=mult  nInputs=2  nOutputs=1  omode=Inherit via internal rule  otype=DataType  scale=constScaleVoltage  floatPrecision=float32_m23  rndmethod=Unbiased  factor=1  satmethod=Symmetric  shift_vec=[0 1 2 -1]  value=0  inPortNames=[' '; ' ';]  outPortNames=[' ']  dspbaimage=dspba_prim.svg  text=fprintf('X');  floatRounding=correct  advOptions=[]  version=20240711
  SampleDelay : DSPBAPrim/SampleDelay  primtype=sampdelay  nInputs=1  nOutputs=1  omode=Inherit via internal rule  otype=sfix(16)  scale=2^-15  floatPrecision=float32_m23  rndmethod=Unbiased  factor=1  satmethod=Symmetric  shift_vec=[0 1 2 -1]  value=1  inPortNames=[' '; ' ';]  outPortNames=[' ']  dspbaimage=dspba_prim.svg  text=dpoly(1, eye(1,value+1), 'z')  flexible=off  slackgroup=0  augmented=0  version=20240711  advOptions=[]
  Sub : DSPBAPrim/Sub  primtype=sub  nInputs=2  nOutputs=1  omode=Inherit via internal rule with word growth  otype=sfix(17)  scale=constScaleVoltage  rndmethod=Unbiased  factor=1  satmethod=Symmetric  shift_vec=[0 1 2 -1]  value=0  inPortNames=['+'; '-';]  outPortNames=[' ']  dspbaimage=dspba_prim.svg  text=fprintf('-');  floatRounding=correct  advOptions=[]  version=20240716
  Sub1 : DSPBAPrim/Sub  primtype=sub  nInputs=2  nOutputs=1  omode=Inherit via internal rule with word growth  otype=sfix(17)  scale=constScaleVoltage  rndmethod=Unbiased  factor=1  satmethod=Symmetric  shift_vec=[0 1 2 -1]  value=0  inPortNames=['+'; '-';]  outPortNames=[' ']  dspbaimage=dspba_prim.svg  text=fprintf('-');  floatRounding=correct  advOptions=[]  version=20240716
  sfix16_0 : DSPBAPrim/Convert  primtype=convert  nInputs=1  nOutputs=1  omode=Specify via dialog  otype=DataType  scale=constScaleVoltage  floatPrecision=float32_m23  rndmethod=Unbiased  factor=1  satmethod=Symmetric  shift_vec=[0 1 2 -1]  value=round([0:255]/17)  inPortNames=[' '; ' ';]  outPortNames=[' '; 'c']  dspbaimage=dspba_prim_wide.svg  text=fprintf('convert');  clipdetect=off  advOptions=[]  version=20240711
  sfix16_1 : DSPBAPrim/Convert  primtype=convert  nInputs=1  nOutputs=1  omode=Specify via dialog  otype=DataType  scale=constScaleVoltage  floatPrecision=float32_m23  rndmethod=Unbiased  factor=1  satmethod=Symmetric  shift_vec=[0 1 2 -1]  value=round([0:255]/17)  inPortNames=[' '; ' ';]  outPortNames=[' '; 'c']  dspbaimage=dspba_prim_wide.svg  text=fprintf('convert');  clipdetect=off  advOptions=[]  version=20240711
  sfix16_2 : DSPBAPrim/Convert  primtype=convert  nInputs=1  nOutputs=1  omode=Specify via dialog  otype=DataType  scale=constScaleVoltage  floatPrecision=float32_m23  rndmethod=Unbiased  factor=1  satmethod=Symmetric  shift_vec=[0 1 2 -1]  value=round([0:255]/17)  inPortNames=[' '; ' ';]  outPortNames=[' '; 'c']  dspbaimage=dspba_prim_wide.svg  text=fprintf('convert');  clipdetect=off  advOptions=[]  version=20240711
  sfix16_3 : DSPBAPrim/Convert  primtype=convert  nInputs=1  nOutputs=1  omode=Specify via dialog  otype=sfix(26)  scale=2^-20  floatPrecision=float32_m23  rndmethod=Unbiased  factor=1  satmethod=Symmetric  shift_vec=[0 1 2 -1]  value=round([0:255]/17)  inPortNames=[' '; ' ';]  outPortNames=[' '; 'c']  dspbaimage=dspba_prim_wide.svg  text=fprintf('convert');  clipdetect=off  advOptions=[]  version=20240711
  sfix16_5 : DSPBAPrim/Convert  primtype=convert  nInputs=1  nOutputs=1  omode=Specify via dialog  otype=DataType_Current  scale=constScale_Current  floatPrecision=float32_m23  rndmethod=Unbiased  factor=1  satmethod=Symmetric  shift_vec=[0 1 2 -1]  value=round([0:255]/17)  inPortNames=[' '; ' ';]  outPortNames=[' '; 'c']  dspbaimage=dspba_prim_wide.svg  text=fprintf('convert');  clipdetect=off  advOptions=[]  version=20240711
  speed - sfix16_En6_2 : DSPBAPrim/Convert  primtype=convert  nInputs=1  nOutputs=1  omode=Specify via dialog  otype=DataTypeCurrentDerivative  scale=constScaleCurrentDerivative  floatPrecision=float32_m23  rndmethod=Unbiased  factor=1  satmethod=Symmetric  shift_vec=[0 1 2 -1]  value=round([0:255]/17)  inPortNames=[' '; ' ';]  outPortNames=[' '; 'c']  dspbaimage=dspba_prim_wide.svg  text=fprintf('convert');  clipdetect=off  advOptions=[]  version=20240711
  di_dt_A_s : Outport
  i_A_k : Outport  Port=2
  wires:
  vBemf_V/1 -> Sub1/2
  v_V/1 -> Sub/1
  i_A_k_1/1 -> Mult2/1
  inv_Lphase_H/1 -> Mult1/2
  Rphase_ohm/1 -> Mult2/2
  SampleTime_s/1 -> Mult/2
  Mult/1 -> sfix16_3/1
  Add/1 -> sfix16_5/1
  Mult2/1 -> sfix16_0/1
  Sub/1 -> sfix16_1/1
  Sub1/1 -> sfix16_2/1
  Mult1/1 -> speed - sfix16_En6_2/1
  sfix16_0/1 -> Sub/2
  sfix16_1/1 -> Sub1/1
  sfix16_3/1 -> Add/1
  sfix16_5/1 -> SampleDelay/1, i_A_k/1
  speed - sfix16_En6_2/1 -> di_dt_A_s/1, Mult/1
  sfix16_2/1 -> Mult1/1
  SampleDelay/1 -> Add/2

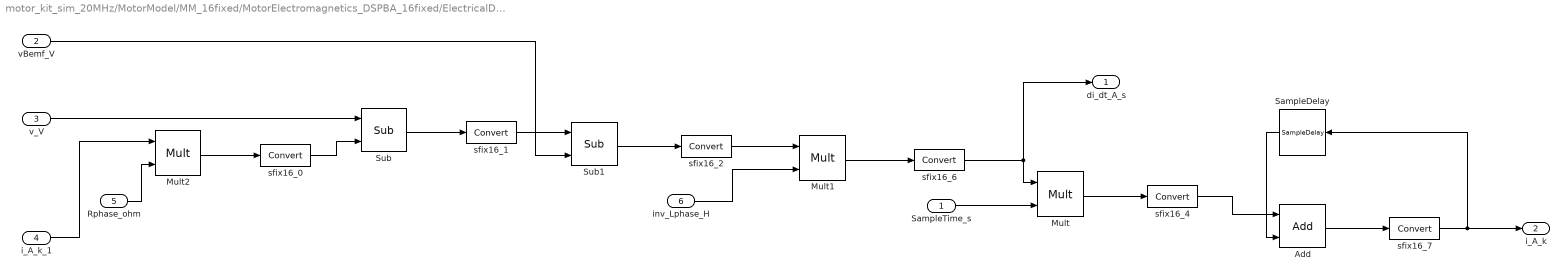
== system motor_kit_sim_20MHz/MotorModel/MM_16fixed/MotorElectromagnetics_DSPBA_16fixed/ElectricalDynamicsDSPBA_16fixed/ElectricalDynamicsOnePhase_Beta_DSPBA16fixed ==
  SampleTime_s : Inport
  vBemf_V : Inport  Port=2
  v_V : Inport  Port=3
  i_A_k_1 : Inport  Port=4
  Rphase_ohm : Inport  Port=5
  inv_Lphase_H : Inport  Port=6
  Add : DSPBAPrim/Add  primtype=add  nInputs=evalAionMaskParam(gcb,'value',1)  nOutputs=1  omode=Inherit via internal rule with word growth  otype=sfix(17)  scale=constScaleCurrent  rndmethod=Unbiased  factor=1  satmethod=Symmetric  shift_vec=[0 1 2 -1]  value=2  inPortNames=[' '; ' ';]  outPortNames=[' ']  dspbaimage=dspba_prim.svg  text=fprintf('+');  genFPC=off  floatRounding=correct  advOptions=[]  version=20240716
  Mult : DSPBAPrim/Mult  primtype=mult  nInputs=2  nOutputs=1  omode=Inherit via internal rule  otype=sfix(64)  scale=2^-34  floatPrecision=float32_m23  rndmethod=Unbiased  factor=1  satmethod=Symmetric  shift_vec=[0 1 2 -1]  value=0  inPortNames=[' '; ' ';]  outPortNames=[' ']  dspbaimage=dspba_prim.svg  text=fprintf('X');  floatRounding=correct  advOptions=[]  version=20240711
  Mult1 : DSPBAPrim/Mult  primtype=mult  nInputs=2  nOutputs=1  omode=Inherit via internal rule  otype=DataType  scale=constScaleCurrentDerivative  floatPrecision=float32_m23  rndmethod=Unbiased  factor=1  satmethod=Symmetric  shift_vec=[0 1 2 -1]  value=0  inPortNames=[' '; ' ';]  outPortNames=[' ']  dspbaimage=dspba_prim.svg  text=fprintf('X');  floatRounding=correct  advOptions=[]  version=20240711
  Mult2 : DSPBAPrim/Mult  primtype=mult  nInputs=2  nOutputs=1  omode=Inherit via internal rule  otype=DataType  scale=constScaleVoltage  floatPrecision=float32_m23  rndmethod=Unbiased  factor=1  satmethod=Symmetric  shift_vec=[0 1 2 -1]  value=0  inPortNames=[' '; ' ';]  outPortNames=[' ']  dspbaimage=dspba_prim.svg  text=fprintf('X');  floatRounding=correct  advOptions=[]  version=20240711
  SampleDelay : DSPBAPrim/SampleDelay  primtype=sampdelay  nInputs=1  nOutputs=1  omode=Inherit via internal rule  otype=sfix(16)  scale=2^-15  floatPrecision=float32_m23  rndmethod=Unbiased  factor=1  satmethod=Symmetric  shift_vec=[0 1 2 -1]  value=1  inPortNames=[' '; ' ';]  outPortNames=[' ']  dspbaimage=dspba_prim.svg  text=dpoly(1, eye(1,value+1), 'z')  flexible=off  slackgroup=0  augmented=0  version=20240711  advOptions=[]
  Sub : DSPBAPrim/Sub  primtype=sub  nInputs=2  nOutputs=1  omode=Inherit via internal rule with word growth  otype=DataType  scale=constScaleVoltage  rndmethod=Unbiased  factor=1  satmethod=Symmetric  shift_vec=[0 1 2 -1]  value=0  inPortNames=['+'; '-';]  outPortNames=[' ']  dspbaimage=dspba_prim.svg  text=fprintf('-');  floatRounding=correct  advOptions=[]  version=20240716
  Sub1 : DSPBAPrim/Sub  primtype=sub  nInputs=2  nOutputs=1  omode=Inherit via internal rule with word growth  otype=sfix(17)  scale=constScaleVoltage  rndmethod=Unbiased  factor=1  satmethod=Symmetric  shift_vec=[0 1 2 -1]  value=0  inPortNames=['+'; '-';]  outPortNames=[' ']  dspbaimage=dspba_prim.svg  text=fprintf('-');  floatRounding=correct  advOptions=[]  version=20240716
  sfix16_0 : DSPBAPrim/Convert  primtype=convert  nInputs=1  nOutputs=1  omode=Specify via dialog  otype=DataType  scale=constScaleVoltage  floatPrecision=float32_m23  rndmethod=Unbiased  factor=1  satmethod=Symmetric  shift_vec=[0 1 2 -1]  value=round([0:255]/17)  inPortNames=[' '; ' ';]  outPortNames=[' '; 'c']  dspbaimage=dspba_prim_wide.svg  text=fprintf('convert');  clipdetect=off  advOptions=[]  version=20240711
  sfix16_1 : DSPBAPrim/Convert  primtype=convert  nInputs=1  nOutputs=1  omode=Specify via dialog  otype=DataType  scale=constScaleVoltage  floatPrecision=float32_m23  rndmethod=Unbiased  factor=1  satmethod=Symmetric  shift_vec=[0 1 2 -1]  value=round([0:255]/17)  inPortNames=[' '; ' ';]  outPortNames=[' '; 'c']  dspbaimage=dspba_prim_wide.svg  text=fprintf('convert');  clipdetect=off  advOptions=[]  version=20240711
  sfix16_2 : DSPBAPrim/Convert  primtype=convert  nInputs=1  nOutputs=1  omode=Specify via dialog  otype=DataType  scale=constScaleVoltage  floatPrecision=float32_m23  rndmethod=Unbiased  factor=1  satmethod=Symmetric  shift_vec=[0 1 2 -1]  value=round([0:255]/17)  inPortNames=[' '; ' ';]  outPortNames=[' '; 'c']  dspbaimage=dspba_prim_wide.svg  text=fprintf('convert');  clipdetect=off  advOptions=[]  version=20240711
  sfix16_4 : DSPBAPrim/Convert  primtype=convert  nInputs=1  nOutputs=1  omode=Specify via dialog  otype=sfix(26)  scale=2^-20  floatPrecision=float32_m23  rndmethod=Unbiased  factor=1  satmethod=Symmetric  shift_vec=[0 1 2 -1]  value=round([0:255]/17)  inPortNames=[' '; ' ';]  outPortNames=[' '; 'c']  dspbaimage=dspba_prim_wide.svg  text=fprintf('convert');  clipdetect=off  advOptions=[]  version=20240711
  sfix16_6 : DSPBAPrim/Convert  primtype=convert  nInputs=1  nOutputs=1  omode=Specify via dialog  otype=DataTypeCurrentDerivative  scale=constScaleCurrentDerivative  floatPrecision=float32_m23  rndmethod=Unbiased  factor=1  satmethod=Symmetric  shift_vec=[0 1 2 -1]  value=round([0:255]/17)  inPortNames=[' '; ' ';]  outPortNames=[' '; 'c']  dspbaimage=dspba_prim_wide.svg  text=fprintf('convert');  clipdetect=off  advOptions=[]  version=20240711
  sfix16_7 : DSPBAPrim/Convert  primtype=convert  nInputs=1  nOutputs=1  omode=Specify via dialog  otype=DataType_Current  scale=constScale_Current  floatPrecision=float32_m23  rndmethod=Unbiased  factor=1  satmethod=Symmetric  shift_vec=[0 1 2 -1]  value=round([0:255]/17)  inPortNames=[' '; ' ';]  outPortNames=[' '; 'c']  dspbaimage=dspba_prim_wide.svg  text=fprintf('convert');  clipdetect=off  advOptions=[]  version=20240711
  di_dt_A_s : Outport
  i_A_k : Outport  Port=2
  wires:
  Sub1/1 -> sfix16_2/1
  Sub/1 -> sfix16_1/1
  Mult2/1 -> sfix16_0/1
  Add/1 -> sfix16_7/1
  Mult/1 -> sfix16_4/1
  SampleTime_s/1 -> Mult/2
  Mult1/1 -> sfix16_6/1
  Rphase_ohm/1 -> Mult2/2
  inv_Lphase_H/1 -> Mult1/2
  i_A_k_1/1 -> Mult2/1
  v_V/1 -> Sub/1
  vBemf_V/1 -> Sub1/2
  sfix16_0/1 -> Sub/2
  sfix16_1/1 -> Sub1/1
  sfix16_2/1 -> Mult1/1
  sfix16_4/1 -> Add/1
  sfix16_6/1 -> Mult/1, di_dt_A_s/1
  sfix16_7/1 -> SampleDelay/1, i_A_k/1
  SampleDelay/1 -> Add/2

== system motor_kit_sim_20MHz/MotorModel/MM_16fixed/MotorElectromagnetics_DSPBA_16fixed/inv_Clarke_16fixed/Subsystem1 ==
  In1 : Inport
  Const3 : DSPBAPrim/Const  primtype=const  nInputs=0  nOutputs=1  omode=Specify via dialog  otype=DataType  scale=2^-15  floatPrecision=float32_m23  rndmethod=Unbiased  factor=1  satmethod=Symmetric  shift_vec=[0 1 2 -1]  value=constVal  inPortNames=['+'; '+';]  outPortNames=[' ']  dspbaimage=dspba_prim.svg  text=fprintf('%s', num2str(value));  warnSaturation=on  version=20240711  SampleTime=inf
  Mult1 : DSPBAPrim/Mult  primtype=mult  nInputs=2  nOutputs=1  omode=Inherit via internal rule  otype=DataType  scale=constScaleCurrent  floatPrecision=float32_m23  rndmethod=Unbiased  factor=1  satmethod=Symmetric  shift_vec=[0 1 2 -1]  value=0  inPortNames=[' '; ' ';]  outPortNames=[' ']  dspbaimage=dspba_prim.svg  text=fprintf('X');  floatRounding=correct  advOptions=[]  version=20240711
  Out1 : Outport
  wires:
  Const3/1 -> Mult1/2
  Mult1/1 -> Out1/1
  In1/1 -> Mult1/1

== system motor_kit_sim_20MHz/MotorModel/MM_16fixed/MotorElectromagnetics_DSPBA_16fixed/inv_Clarke_16fixed/Subsystem4 ==
  In1 : Inport
  Const3 : DSPBAPrim/Const  primtype=const  nInputs=0  nOutputs=1  omode=Specify via dialog  otype=ufix(16)  scale=2^-15  floatPrecision=float32_m23  rndmethod=Unbiased  factor=1  satmethod=Symmetric  shift_vec=[0 1 2 -1]  value=constVal  inPortNames=['+'; '+';]  outPortNames=[' ']  dspbaimage=dspba_prim.svg  text=fprintf('%s', num2str(value));  warnSaturation=on  version=20240711  SampleTime=inf
  Mult1 : DSPBAPrim/Mult  primtype=mult  nInputs=2  nOutputs=1  omode=Inherit via internal rule  otype=DataType  scale=constScaleCurrent  floatPrecision=float32_m23  rndmethod=Unbiased  factor=1  satmethod=Symmetric  shift_vec=[0 1 2 -1]  value=0  inPortNames=[' '; ' ';]  outPortNames=[' ']  dspbaimage=dspba_prim.svg  text=fprintf('X');  floatRounding=correct  advOptions=[]  version=20240711
  Out1 : Outport
  wires:
  Const3/1 -> Mult1/2
  Mult1/1 -> Out1/1
  In1/1 -> Mult1/1

== system motor_kit_sim_20MHz/MotorModel/MM_16fixed/MotorElectromagnetics_DSPBA_16fixed/inv_Clarke_16fixed/Subsystem5 ==
  In1 : Inport
  Const3 : DSPBAPrim/Const  primtype=const  nInputs=0  nOutputs=1  omode=Specify via dialog  otype=DataType  scale=2^-15  floatPrecision=float32_m23  rndmethod=Unbiased  factor=1  satmethod=Symmetric  shift_vec=[0 1 2 -1]  value=constVal  inPortNames=['+'; '+';]  outPortNames=[' ']  dspbaimage=dspba_prim.svg  text=fprintf('%s', num2str(value));  warnSaturation=on  version=20240711  SampleTime=inf
  Mult1 : DSPBAPrim/Mult  primtype=mult  nInputs=2  nOutputs=1  omode=Inherit via internal rule  otype=DataType  scale=constScaleCurrent  floatPrecision=float32_m23  rndmethod=Unbiased  factor=1  satmethod=Symmetric  shift_vec=[0 1 2 -1]  value=0  inPortNames=[' '; ' ';]  outPortNames=[' ']  dspbaimage=dspba_prim.svg  text=fprintf('X');  floatRounding=correct  advOptions=[]  version=20240711
  Out1 : Outport
  wires:
  In1/1 -> Mult1/1
  Mult1/1 -> Out1/1
  Const3/1 -> Mult1/2

== system motor_kit_sim_20MHz/MotorModel/MM_16fixed/MotorElectromagnetics_DSPBA_16fixed/sine_cosine_16fixed/modulus ==
  In1 : Inport
  Convert1 : DSPBAPrim/Convert  primtype=convert  nInputs=1  nOutputs=1  omode=Specify via dialog  otype=ufix(16)  scale=2^-16  floatPrecision=float32_m23  rndmethod=TruncateToZero  factor=1  satmethod=None  shift_vec=[0 1 2 -1]  value=round([0:255]/17)  inPortNames=[' '; ' ';]  outPortNames=[' '; 'c']  dspbaimage=dspba_prim_wide.svg  text=fprintf('convert');  clipdetect=off  advOptions=[]  version=20240711
  Convert2 : DSPBAPrim/Convert  primtype=convert  nInputs=1  nOutputs=1  omode=Specify via dialog  otype=ufix(16)  scale=1  floatPrecision=float32_m23  rndmethod=TruncateToZero  factor=1  satmethod=None  shift_vec=[0 1 2 -1]  value=round([0:255]/17)  inPortNames=[' '; ' ';]  outPortNames=[' '; 'c']  dspbaimage=dspba_prim_wide.svg  text=fprintf('convert');  clipdetect=off  advOptions=[]  version=20240711
  Sub1 : DSPBAPrim/Sub  primtype=sub  nInputs=2  nOutputs=1  omode=Inherit via internal rule  otype=ufix(16)  scale=2^-14  rndmethod=Unbiased  factor=1  satmethod=Symmetric  shift_vec=[0 1 2 -1]  value=0  inPortNames=['+'; '-';]  outPortNames=[' ']  dspbaimage=dspba_prim.svg  text=fprintf('-');  floatRounding=correct  advOptions=[]  version=20240716
  Out1 : Outport
  wires:
  Convert2/1 -> Sub1/2  "integer_part"
  In1/1 -> Convert2/1, Sub1/1  "phi"
  Sub1/1 -> Convert1/1  "modulus"
  Convert1/1 -> Out1/1
